simulink model "s06_sig_template"  (R2025a)
settings: Solver=ode4  StartTime=0.0  StopTime=inf  FixedStep=P_sim_dt  RelTol=1e-3  EnableMultiTasking=on
InitFcn:
  | s06_data;
values from neighbouring files (symbols this model uses):
  CarInputsCmdForward = uint8(1)    [i01_data.m]
  ManeuverTypePark = uint8(1)    [i01_data.m]
  ManeuverTypePathFollow = uint8(3)    [i01_data.m]
  P_c_locate_problist = ones(P_car_cnt, 1, 'single')    [s06_data.m]
  P_cpseq = Simulink.Bus.createMATLABStruct('CHECKPOINTSEQUENCEMSG', [])    [i01_data.m]
  P_display_dt = 50e-3    (= 0.05)    [s06_data.m]
  P_dt = 25e-3    (= 0.025)    [s06_data.m]
  P_p_deltan_max = 1    [d01_data.m]    (also in d71_data.m = 0.93)
  P_p_deltan_min = -P_p_deltan_max    (= -1)    [d01_data.m]    (also in d71_data.m = -0.93)
  P_p_un_max = 1    [d01_data.m]    (also in d71_data.m = 0.2)
  P_p_un_min = -P_p_un_max    (= -1)    [d01_data.m]    (also in d71_data.m = -0.2)
  P_p_xvec0 = [ P_p_v0; P_p_s10; P_p_s20; P_p_psi0; 0; 0; 0 ]    [d01_data.m]    (also in d71_data.m)
  P_p_xvec1 = [ P_p_v0; P_p_s11; P_p_s21; P_p_psi1; 0; 0; 0 ]    [d01_data.m]    (also in d71_data.m)
  P_vfilter = single([ 0.0 0.0 ... (first row only)    [s06_data.m]
undefined symbols (not defined in the file or in its folder): mbc_car_display, P_p, P_track
libraries: vrlib x2
settings Model: Creator=ftraenkle  LastModifiedBy=ftraenkle
settings SolverCC: AlgebraicLoopSolver=TrustRegion
settings DataIOCC: LimitDataPoints=on  InspectSignalLogs=on  ReturnWorkspaceOutputs=off
settings OptimizationCC: DefaultParameterBehavior=Inlined  EnhancedBackFolding=on  PassReuseOutputArgsAs=Individual arguments  ExpressionDepthLimit=2147483647.0  ZeroExternalMemoryAtStartup=off  ZeroInternalMemoryAtStartup=off  OptimizeBlockOrder=speed  DifferentSizesBufferReuse=on  OptimizationCustomize=off  EfficientTunableParamExpr=on
settings DebuggingCC: MergeDetectMultiDrivingBlocksExec=none  SolverPrmCheckMsg=warning  ParameterTunabilityLossMsg=error  UnconnectedInputMsg=warning  UnconnectedOutputMsg=warning  UnconnectedLineMsg=warning  BusObjectLabelMismatch=error  AllowSymbolicDim=off  StateNameClashWarn=warning  SFUnexpectedBacktrackingDiag=warning  SFNoUnconditionalDefaultTransitionDiag=warning  SFExecutionAtInitializationDiag=none  ArithmeticOperatorsInVariantConditions=warning
settings HardwareCC: ProdBitPerLong=64.0  ProdHWDeviceType=Intel->x86-64 (Linux 64)
settings ModelReferenceCC: EnableRefExpFcnMdlSchedulingChecks=on  PropagateSignalLabelsOutOfModel=off
settings SFSimCC: SimUseLocalCustomCode=off  CustomCodeUndefinedFunction=UseInterfaceOnly
settings RTWCC: SystemTargetFile=ert.tlc  GenCodeOnly=on  PackageGeneratedCodeAndArtifacts=on  PackageName=d1.zip  TemplateMakefile=ert_default_tmf  GenerateReport=on  RTWUseLocalCustomCode=off  IncludeHyperlinkInReport=on  GenerateTraceInfo=on  GenerateTraceReportEml=on  GPUComputeCapability=3.5  DLArmComputeVersion=19.05  Description=Embedded Coder
settings CodeAppCC: ForceParamTrailComments=on  IgnoreCustomStorageClasses=off  OperatorAnnotations=on  SimulinkDataObjDesc=on  SFDataObjDesc=on  InsertBlockDesc=on
settings ERTTargetCC: ExtModeTransport=0.0  ExtModeStaticAlloc=off  ExtModeMexFile=ext_comm  ExtModeIntrfLevel=Level1  RootIOFormat=Structure reference  ERTCustomFileTemplate=example_file_process.tlc  DynamicArrayContainerType=coder::array  TargetLangStandard=C99 (ISO)  SupportVariableSizeSignals=on
settings ConfigComp: CovMetricSettings=dw  CovSaveCumulativeToWorkspaceVar=on  CovSaveSingleToWorkspaceVar=on  CovExternalEMLEnable=off

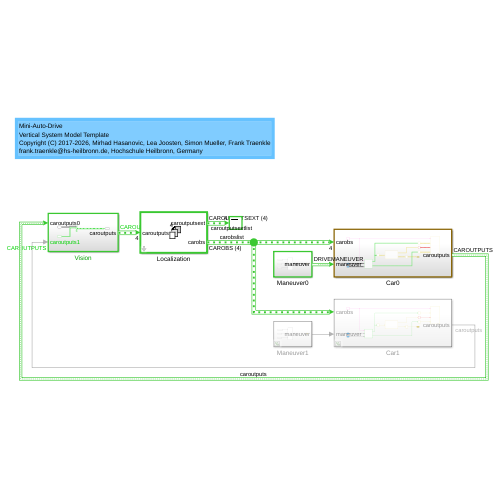
[thumbnail: Simulink's stored preview of the top-level diagram]
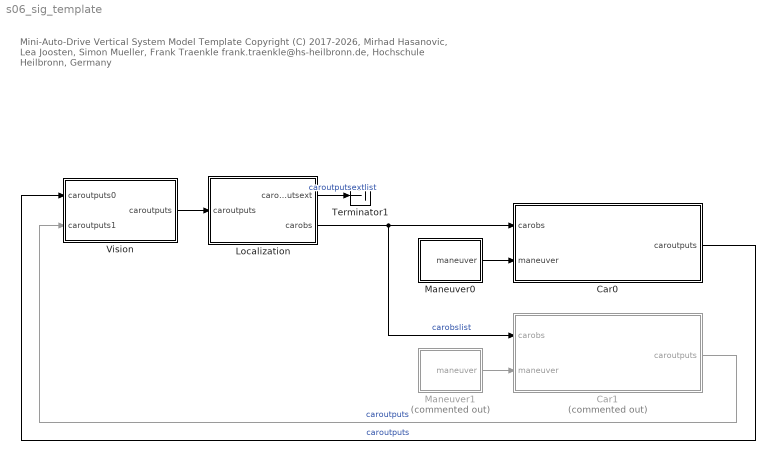
== system s06_sig_template ==
  note: Mini-Auto-Drive
      | Vertical System Model Template
      | Copyright (C) 2017-2026, Mirhad Hasanovic, Lea Joosten, Simon Mueller, Frank Traenkle
      | frank.traenkle@hs-heilbronn.de, Hochschule Heilbronn, Germany
  Car0 : Subsystem
  Car1 : Subsystem  Commented=on
  Localization : Subsystem  TreatAsAtomicUnit=on  mask{P_mask_problist=P_c_locate_problist}
      mask prompts: P_mask_problist "Locate Probability"
  Maneuver0 : Subsystem
  Maneuver1 : Subsystem  Commented=on
  Terminator1 : Terminator
  Vision : Subsystem
  wires:
  Car0/1(caroutputs) -> Vision/1(caroutputs0)  "caroutputs"
  Localization/2(carobs) -> Car1/1(carobs), Car0/1(carobs)  "carobslist"
  Vision/1(caroutputs) -> Localization/1(caroutputs)
  Car1/1(caroutputs) -> Vision/2(caroutputs1)  "caroutputs"
  Maneuver0/1(maneuver) -> Car0/2(maneuver)
  Maneuver1/1(maneuver) -> Car1/2(maneuver)
  Localization/1(caroutputsext) -> Terminator1/1  "caroutputsextlist"

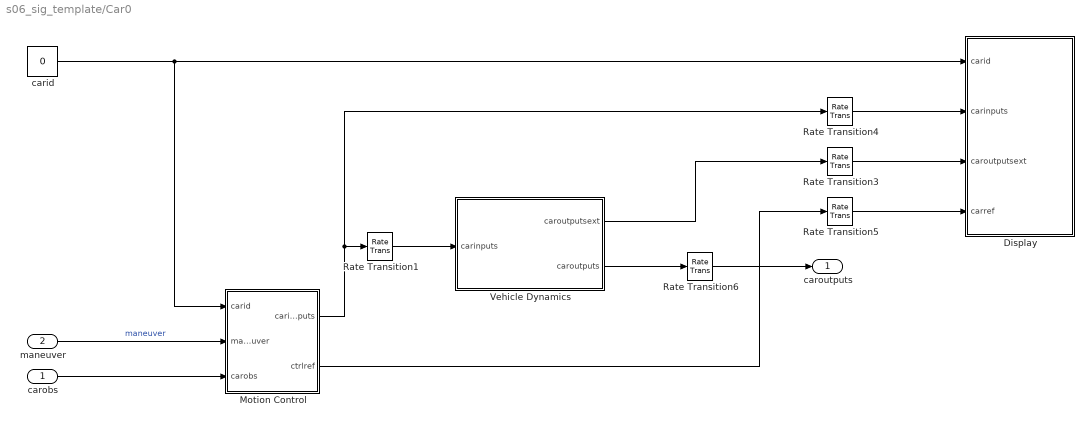
== system s06_sig_template/Car0 ==
  carobs : Inport  OutDataTypeStr=Bus: CAROBS
  maneuver : Inport  Port=2
  Display : Subsystem  TreatAsAtomicUnit=on  SystemSampleTime=P_display_dt
  Motion Control : Subsystem  TreatAsAtomicUnit=on  SystemSampleTime=P_dt
  Rate Transition1 : RateTransition  Integrity=off
  Rate Transition{3..6} (4 alike) : RateTransition
  Vehicle Dynamics : Subsystem  mask{P_mask_vec0=P_p_xvec0, P_mask_p=P_p(1)}
      mask prompts: P_mask_vec0 "Initial value"; P_mask_p "Parameters"
  carid : Constant  Value=0
  caroutputs : Outport  OutDataTypeStr=Bus: CAROUTPUTS
  wires:
  Vehicle Dynamics/1(caroutputsext) -> Rate Transition3/1
  Rate Transition5/1 -> Display/4(carref)
  Rate Transition3/1 -> Display/3(caroutputsext)
  Rate Transition4/1 -> Display/2(carinputs)
  Rate Transition1/1 -> Vehicle Dynamics/1(carinputs)
  Vehicle Dynamics/2(caroutputs) -> Rate Transition6/1
  Rate Transition6/1 -> caroutputs/1
  carid/1 -> Motion Control/1(carid), Display/1(carid)
  Motion Control/1(carinputs) -> Rate Transition4/1, Rate Transition1/1
  Motion Control/2(ctrlref) -> Rate Transition5/1
  carobs/1 -> Motion Control/3(carobs)
  maneuver/1 -> Motion Control/2(maneuver)  "maneuver"

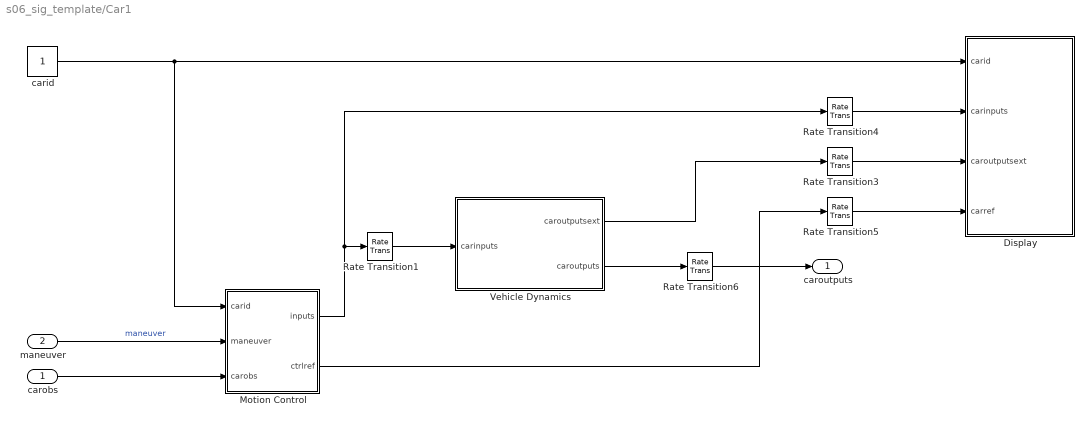
== system s06_sig_template/Car1 ==
  carobs : Inport  OutDataTypeStr=Bus: CAROBS
  maneuver : Inport  Port=2
  Display : Subsystem  TreatAsAtomicUnit=on  SystemSampleTime=P_display_dt
  Motion Control : Subsystem  TreatAsAtomicUnit=on  SystemSampleTime=P_dt
  Rate Transition{1,3..6} (5 alike) : RateTransition
  Vehicle Dynamics : Subsystem  mask{P_mask_vec0=P_p_xvec1, P_mask_p=P_p(1)}
      mask prompts: P_mask_vec0 "Initial value"; P_mask_p "Parameters"
  carid : Constant
  caroutputs : Outport  OutDataTypeStr=Bus: CAROUTPUTS
  wires:
  Vehicle Dynamics/1(caroutputsext) -> Rate Transition3/1
  Rate Transition5/1 -> Display/4(carref)
  Rate Transition3/1 -> Display/3(caroutputsext)
  Rate Transition4/1 -> Display/2(carinputs)
  Rate Transition1/1 -> Vehicle Dynamics/1(carinputs)
  Vehicle Dynamics/2(caroutputs) -> Rate Transition6/1
  Rate Transition6/1 -> caroutputs/1
  carid/1 -> Motion Control/1(carid), Display/1(carid)
  Motion Control/1(inputs) -> Rate Transition4/1, Rate Transition1/1
  Motion Control/2(ctrlref) -> Rate Transition5/1
  carobs/1 -> Motion Control/3(carobs)
  maneuver/1 -> Motion Control/2(maneuver)  "maneuver"

== system s06_sig_template/Localization ==
  caroutputs : Inport  Partition=on  PartitionDimension=1  PartitionWidth=1  PartitionOffset=0
  Constant : Constant  Value=true
  For Each : ForEach  DisableCoverage=on  IterateSubsysMaskParameter=on
  Locate : Subsystem
  caroutputsext : Outport  ConcatenationDimension=1
  carobs : Outport  Port=2  ConcatenationDimension=1
  wires:
  Locate/1(caroutputsext) -> caroutputsext/1
  Constant/1 -> Locate/Enable
  caroutputs/1 -> Locate/1(caroutputs)
  Locate/2(carobs) -> carobs/1

== system s06_sig_template/Maneuver0 ==
  Constant : Constant  Value=ManeuverTypePark
  Constant1 : Constant  Value=single(0.5)
  Constant2 : Constant  Value=single(2.0)
  Create Maneuver : MATLAB Function  TreatAsAtomicUnit=on
  maneuver : Outport
  wires:
  Constant/1 -> Create Maneuver/1(type)
  Constant1/1 -> Create Maneuver/2(vmax)
  Constant2/1 -> Create Maneuver/3(xref)
  Create Maneuver/1(maneuver) -> maneuver/1  "maneuver"

== system s06_sig_template/Maneuver1 ==
  Constant : Constant  Value=ManeuverTypePathFollow
  Constant1 : Constant  Value=single(0.5)
  Constant2 : Constant  Value=single(1.0)
  Create Maneuver : MATLAB Function  TreatAsAtomicUnit=on
  maneuver : Outport
  wires:
  Create Maneuver/1(maneuver) -> maneuver/1  "maneuver"
  Constant2/1 -> Create Maneuver/3(xref)
  Constant1/1 -> Create Maneuver/2(vmax)
  Constant/1 -> Create Maneuver/1(type)

== system s06_sig_template/Vision ==
  caroutputs0 : Inport  OutDataTypeStr=Bus:CAROUTPUTS
  caroutputs1 : Inport  Port=2  OutDataTypeStr=Bus:CAROUTPUTS
  Vector Concatenate : Concatenate  NumInputs=P_car_cnt
  caroutputs : Outport  OutDataTypeStr=Bus:CAROUTPUTS
  wires:
  Vector Concatenate/1 -> caroutputs/1  "caroutputs"
  caroutputs0/1 -> Vector Concatenate/1
  caroutputs1/1 -> Vector Concatenate/2

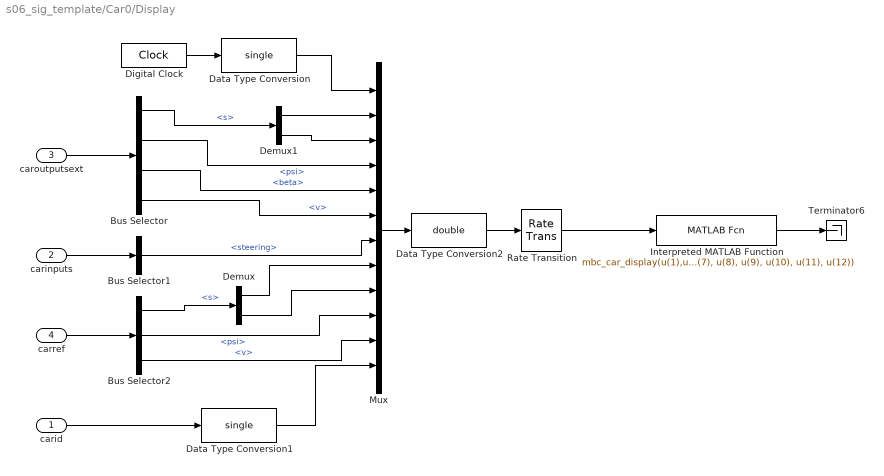
== system s06_sig_template/Car0/Display ==
  carid : Inport
  carinputs : Inport  Port=2
  caroutputsext : Inport  Port=3
  carref : Inport  Port=4
  Bus Selector : BusSelector  OutputSignals=s,psi,beta,v
  Bus Selector1 : BusSelector  OutputSignals=steering
  Bus Selector2 : BusSelector  OutputSignals=s,psi,v
  Data Type Conversion : DataTypeConversion  OutDataTypeStr=single  SaturateOnIntegerOverflow=off  RndMeth=Floor
  Data Type Conversion1 : DataTypeConversion  OutDataTypeStr=single  SaturateOnIntegerOverflow=off  RndMeth=Floor
  Data Type Conversion2 : DataTypeConversion  OutDataTypeStr=double  SaturateOnIntegerOverflow=off  RndMeth=Floor
  Demux : Demux  Outputs=2
  Demux1 : Demux  Outputs=2
  Digital Clock : DigitalClock  SampleTime=-1
  Interpreted MATLAB Function : MATLABFcn  MATLABFcn=mbc_car_display(u(1),u(2),u(3),u(4),u(5), u(6), u(7), u(8), u(9), u(10), u(11), u(12))
  Mux : Mux  Inputs=12
  Rate Transition : RateTransition  OutPortSampleTime=P_display_dt
  Terminator6 : Terminator
  wires:
  caroutputsext/1 -> Bus Selector/1
  Interpreted MATLAB Function/1 -> Terminator6/1
  Mux/1 -> Data Type Conversion2/1
  Rate Transition/1 -> Interpreted MATLAB Function/1
  Digital Clock/1 -> Data Type Conversion/1
  Bus Selector/2 -> Mux/4  "<psi>"
  carinputs/1 -> Bus Selector1/1
  Bus Selector1/1 -> Mux/7  "<steering>"
  Bus Selector/3 -> Mux/5  "<beta>"
  Bus Selector/4 -> Mux/6  "<v>"
  carref/1 -> Bus Selector2/1
  Bus Selector2/3 -> Mux/11  "<v>"
  Bus Selector2/2 -> Mux/10  "<psi>"
  Bus Selector2/1 -> Demux/1  "<s>"
  carid/1 -> Data Type Conversion1/1
  Data Type Conversion/1 -> Mux/1
  Data Type Conversion1/1 -> Mux/12
  Data Type Conversion2/1 -> Rate Transition/1
  Demux/1 -> Mux/8
  Demux/2 -> Mux/9
  Bus Selector/1 -> Demux1/1  "<s>"
  Demux1/1 -> Mux/2
  Demux1/2 -> Mux/3

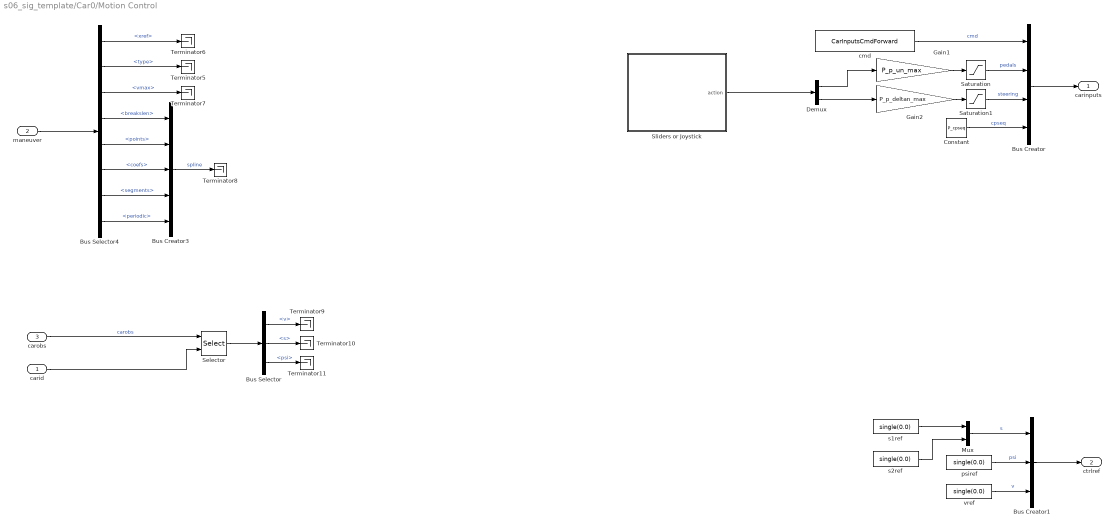
== system s06_sig_template/Car0/Motion Control ==
  carid : Inport
  maneuver : Inport  Port=2
  carobs : Inport  Port=3
  Bus Creator : BusCreator  Inputs=4  OutDataTypeStr=Bus: CARINPUTS  NonVirtualBus=on
  Bus Creator1 : BusCreator  Inputs=3  OutDataTypeStr=Bus: CTRLREFERENCE  NonVirtualBus=on
  Bus Creator3 : BusCreator  Inputs=5  OutDataTypeStr=Bus: SPLINE
  Bus Selector : BusSelector  OutputSignals=v,s,psi
  Bus Selector4 : BusSelector  OutputSignals=xref,type,vmax,breakslen,points,coefs,segments,periodic
  Constant : Constant  Value=P_cpseq  OutDataTypeStr=Bus: CHECKPOINTSEQUENCEMSG
  Demux : Demux  Outputs=2
  Gain1 : Gain  Gain=P_p_un_max
  Gain2 : Gain  Gain=P_p_deltan_max
  Mux : Mux  Inputs=2
  Saturation : Saturate  UpperLimit=P_p_un_max  LowerLimit=P_p_un_min
  Saturation1 : Saturate  UpperLimit=P_p_deltan_max  LowerLimit=P_p_deltan_min
  Selector : Selector  IndexMode=Zero-based  InputPortWidth=P_car_cnt  IndexOptions=Index vector (port)  Indices=0  OutputSizes=1
  Sliders or Joystick : Subsystem  Variant=on  VariantControlMode=label  LabelModeActiveChoice=true
  Terminator{5..11} (7 alike) : Terminator
  cmd : Constant  Value=CarInputsCmdForward
  psiref : Constant  Value=single(0.0)
  s1ref : Constant  Value=single(0.0)
  s2ref : Constant  Value=single(0.0)
  vref : Constant  Value=single(0.0)
  carinputs : Outport  VectorParamsAs1DForOutWhenUnconnected=off
  ctrlref : Outport  Port=2  VectorParamsAs1DForOutWhenUnconnected=off
  wires:
  Bus Creator1/1 -> ctrlref/1
  vref/1 -> Bus Creator1/3  "v"
  Bus Selector/2 -> Terminator10/1  "<s>"
  Mux/1 -> Bus Creator1/1  "s"
  Bus Selector4/7 -> Bus Creator3/4  "<segments>"
  Bus Selector4/5 -> Bus Creator3/2  "<points>"
  Bus Selector4/6 -> Bus Creator3/3  "<coefs>"
  Bus Selector4/8 -> Bus Creator3/5  "<periodic>"
  Bus Selector4/2 -> Terminator5/1  "<type>"
  Bus Selector4/4 -> Bus Creator3/1  "<breakslen>"
  maneuver/1 -> Bus Selector4/1
  carid/1 -> Selector/2
  carobs/1 -> Selector/1  "carobs"
  Selector/1 -> Bus Selector/1
  Bus Selector4/1 -> Terminator6/1  "<xref>"
  Bus Selector4/3 -> Terminator7/1  "<vmax>"
  Bus Creator3/1 -> Terminator8/1  "spline"
  Bus Selector/1 -> Terminator9/1  "<v>"
  Bus Selector/3 -> Terminator11/1  "<psi>"
  s1ref/1 -> Mux/1
  s2ref/1 -> Mux/2
  psiref/1 -> Bus Creator1/2  "psi"
  Saturation/1 -> Bus Creator/2  "pedals"
  Demux/1 -> Gain1/1
  Constant/1 -> Bus Creator/4  "cpseq"
  Bus Creator/1 -> carinputs/1
  cmd/1 -> Bus Creator/1  "cmd"
  Gain1/1 -> Saturation/1
  Saturation1/1 -> Bus Creator/3  "steering"
  Sliders or Joystick/1(action) -> Demux/1
  Demux/2 -> Gain2/1
  Gain2/1 -> Saturation1/1

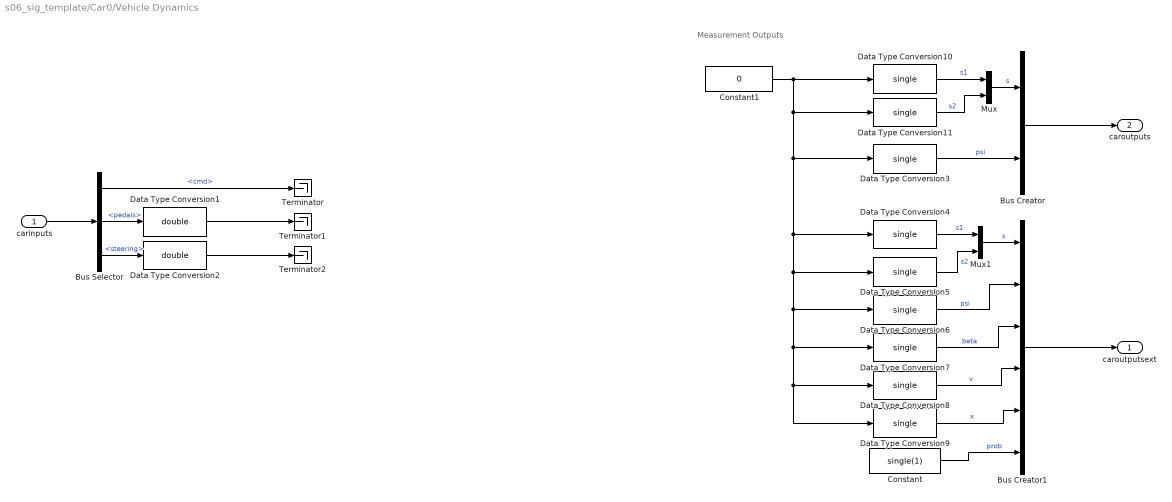
== system s06_sig_template/Car0/Vehicle Dynamics ==
  note: Measurement Outputs
  carinputs : Inport
  Bus Creator : BusCreator  Inputs=2  OutDataTypeStr=Bus: CAROUTPUTS  NonVirtualBus=on
  Bus Creator1 : BusCreator  Inputs=6  OutDataTypeStr=Bus: CAROUTPUTSEXT  NonVirtualBus=on
  Bus Selector : BusSelector  OutputSignals=cmd,pedals,steering
  Constant : Constant  Value=single(1)
  Constant1 : Constant  Value=0
  Data Type Conversion1 : DataTypeConversion  OutDataTypeStr=double  SaturateOnIntegerOverflow=off  RndMeth=Floor
  Data Type Conversion{3..11} (9 alike) : DataTypeConversion  OutDataTypeStr=single  SaturateOnIntegerOverflow=off  RndMeth=Floor
  Data Type Conversion2 : DataTypeConversion  OutDataTypeStr=double  SaturateOnIntegerOverflow=off  RndMeth=Floor
  Mux : Mux  Inputs=2
  Mux1 : Mux  Inputs=2
  Terminator : Terminator
  Terminator1 : Terminator
  Terminator2 : Terminator
  caroutputsext : Outport  OutDataTypeStr=Bus: CAROUTPUTSEXT  VectorParamsAs1DForOutWhenUnconnected=off
  caroutputs : Outport  Port=2  OutDataTypeStr=Bus: CAROUTPUTS  VectorParamsAs1DForOutWhenUnconnected=off
  wires:
  carinputs/1 -> Bus Selector/1
  Bus Selector/2 -> Data Type Conversion1/1  "<pedals>"
  Bus Selector/3 -> Data Type Conversion2/1  "<steering>"
  Bus Creator/1 -> caroutputs/1
  Bus Creator1/1 -> caroutputsext/1
  Bus Selector/1 -> Terminator/1  "<cmd>"
  Data Type Conversion1/1 -> Terminator1/1
  Data Type Conversion2/1 -> Terminator2/1
  Constant1/1 -> Data Type Conversion9/1, Data Type Conversion8/1, Data Type Conversion7/1, Data Type Conversion6/1, Data Type Conversion5/1, Data Type Conversion4/1, Data Type Conversion3/1, Data Type Conversion11/1, Data Type Conversion10/1
  Mux1/1 -> Bus Creator1/1  "s"
  Data Type Conversion5/1 -> Mux1/2  "s2"
  Data Type Conversion4/1 -> Mux1/1  "s1"
  Mux/1 -> Bus Creator/1  "s"
  Data Type Conversion9/1 -> Bus Creator1/5  "x"
  Data Type Conversion8/1 -> Bus Creator1/4  "v"
  Data Type Conversion7/1 -> Bus Creator1/3  "beta"
  Data Type Conversion6/1 -> Bus Creator1/2  "psi"
  Data Type Conversion3/1 -> Bus Creator/2  "psi"
  Data Type Conversion11/1 -> Mux/2  "s2"
  Data Type Conversion10/1 -> Mux/1  "s1"
  Constant/1 -> Bus Creator1/6  "prob"

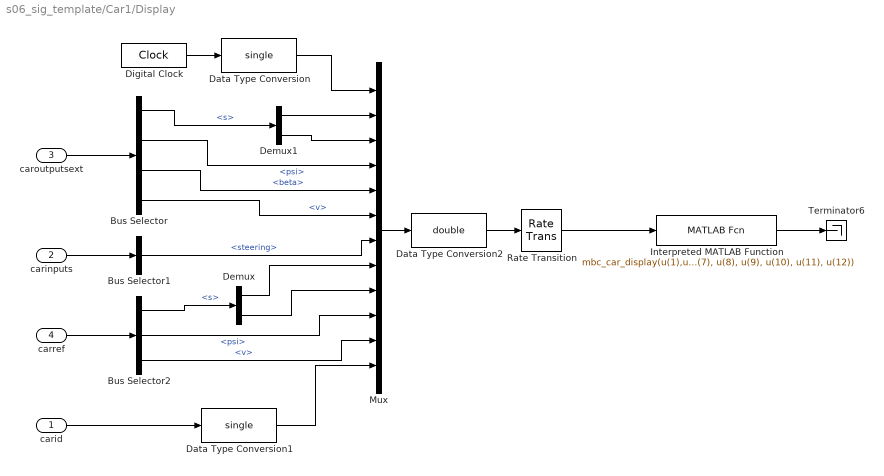
== system s06_sig_template/Car1/Display ==
  carid : Inport
  carinputs : Inport  Port=2
  caroutputsext : Inport  Port=3
  carref : Inport  Port=4
  Bus Selector : BusSelector  OutputSignals=s,psi,beta,v
  Bus Selector1 : BusSelector  OutputSignals=steering
  Bus Selector2 : BusSelector  OutputSignals=s,psi,v
  Data Type Conversion : DataTypeConversion  OutDataTypeStr=single  SaturateOnIntegerOverflow=off  RndMeth=Floor
  Data Type Conversion1 : DataTypeConversion  OutDataTypeStr=single  SaturateOnIntegerOverflow=off  RndMeth=Floor
  Data Type Conversion2 : DataTypeConversion  OutDataTypeStr=double  SaturateOnIntegerOverflow=off  RndMeth=Floor
  Demux : Demux  Outputs=2
  Demux1 : Demux  Outputs=2
  Digital Clock : DigitalClock  SampleTime=-1
  Interpreted MATLAB Function : MATLABFcn  MATLABFcn=mbc_car_display(u(1),u(2),u(3),u(4),u(5), u(6), u(7), u(8), u(9), u(10), u(11), u(12))
  Mux : Mux  Inputs=12
  Rate Transition : RateTransition  OutPortSampleTime=P_display_dt
  Terminator6 : Terminator
  wires:
  caroutputsext/1 -> Bus Selector/1
  Interpreted MATLAB Function/1 -> Terminator6/1
  Mux/1 -> Data Type Conversion2/1
  Rate Transition/1 -> Interpreted MATLAB Function/1
  Digital Clock/1 -> Data Type Conversion/1
  Bus Selector/2 -> Mux/4  "<psi>"
  carinputs/1 -> Bus Selector1/1
  Bus Selector1/1 -> Mux/7  "<steering>"
  Bus Selector/3 -> Mux/5  "<beta>"
  Bus Selector/4 -> Mux/6  "<v>"
  carref/1 -> Bus Selector2/1
  Bus Selector2/3 -> Mux/11  "<v>"
  Bus Selector2/2 -> Mux/10  "<psi>"
  Bus Selector2/1 -> Demux/1  "<s>"
  carid/1 -> Data Type Conversion1/1
  Data Type Conversion/1 -> Mux/1
  Data Type Conversion1/1 -> Mux/12
  Data Type Conversion2/1 -> Rate Transition/1
  Demux/1 -> Mux/8
  Demux/2 -> Mux/9
  Bus Selector/1 -> Demux1/1  "<s>"
  Demux1/1 -> Mux/2
  Demux1/2 -> Mux/3

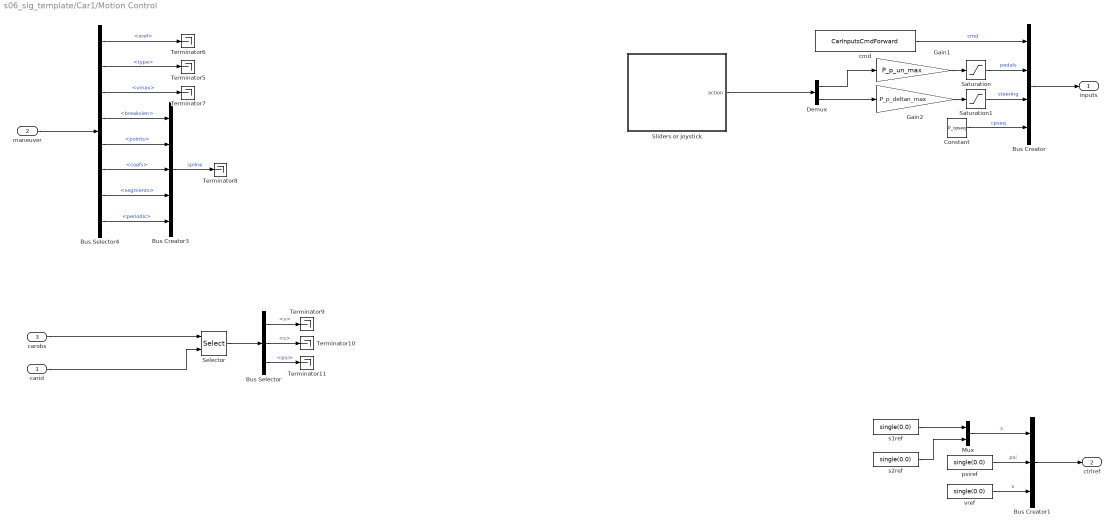
== system s06_sig_template/Car1/Motion Control ==
  carid : Inport
  maneuver : Inport  Port=2
  carobs : Inport  Port=3
  Bus Creator : BusCreator  Inputs=4  OutDataTypeStr=Bus: CARINPUTS  NonVirtualBus=on
  Bus Creator1 : BusCreator  Inputs=3  OutDataTypeStr=Bus: CTRLREFERENCE  NonVirtualBus=on
  Bus Creator3 : BusCreator  Inputs=5  OutDataTypeStr=Bus: SPLINE
  Bus Selector : BusSelector  OutputSignals=v,s,psi
  Bus Selector4 : BusSelector  OutputSignals=xref,type,vmax,breakslen,points,coefs,segments,periodic
  Constant : Constant  Value=P_cpseq  OutDataTypeStr=Bus: CHECKPOINTSEQUENCEMSG
  Demux : Demux  Outputs=2
  Gain1 : Gain  Gain=P_p_un_max
  Gain2 : Gain  Gain=P_p_deltan_max
  Mux : Mux  Inputs=2
  Saturation : Saturate  UpperLimit=P_p_un_max  LowerLimit=P_p_un_min
  Saturation1 : Saturate  UpperLimit=P_p_deltan_max  LowerLimit=P_p_deltan_min
  Selector : Selector  IndexMode=Zero-based  InputPortWidth=P_car_cnt  IndexOptions=Index vector (port)  Indices=0  OutputSizes=1
  Sliders or Joystick : Subsystem  Variant=on  VariantControlMode=label  LabelModeActiveChoice=true
  Terminator{5..11} (7 alike) : Terminator
  cmd : Constant  Value=CarInputsCmdForward
  psiref : Constant  Value=single(0.0)
  s1ref : Constant  Value=single(0.0)
  s2ref : Constant  Value=single(0.0)
  vref : Constant  Value=single(0.0)
  inputs : Outport  VectorParamsAs1DForOutWhenUnconnected=off
  ctrlref : Outport  Port=2  VectorParamsAs1DForOutWhenUnconnected=off
  wires:
  Bus Creator1/1 -> ctrlref/1
  vref/1 -> Bus Creator1/3  "v"
  Bus Selector/2 -> Terminator10/1  "<s>"
  Mux/1 -> Bus Creator1/1  "s"
  Bus Selector4/7 -> Bus Creator3/4  "<segments>"
  Bus Selector4/5 -> Bus Creator3/2  "<points>"
  Bus Selector4/6 -> Bus Creator3/3  "<coefs>"
  Bus Selector4/8 -> Bus Creator3/5  "<periodic>"
  Bus Selector4/2 -> Terminator5/1  "<type>"
  Bus Selector4/4 -> Bus Creator3/1  "<breakslen>"
  maneuver/1 -> Bus Selector4/1
  carid/1 -> Selector/2
  carobs/1 -> Selector/1
  Selector/1 -> Bus Selector/1
  Bus Selector4/1 -> Terminator6/1  "<xref>"
  Bus Selector4/3 -> Terminator7/1  "<vmax>"
  Bus Creator3/1 -> Terminator8/1  "spline"
  Bus Selector/1 -> Terminator9/1  "<v>"
  Bus Selector/3 -> Terminator11/1  "<psi>"
  s1ref/1 -> Mux/1
  s2ref/1 -> Mux/2
  psiref/1 -> Bus Creator1/2  "psi"
  Saturation/1 -> Bus Creator/2  "pedals"
  Demux/1 -> Gain1/1
  Constant/1 -> Bus Creator/4  "cpseq"
  Bus Creator/1 -> inputs/1
  cmd/1 -> Bus Creator/1  "cmd"
  Gain1/1 -> Saturation/1
  Saturation1/1 -> Bus Creator/3  "steering"
  Sliders or Joystick/1(action) -> Demux/1
  Demux/2 -> Gain2/1
  Gain2/1 -> Saturation1/1

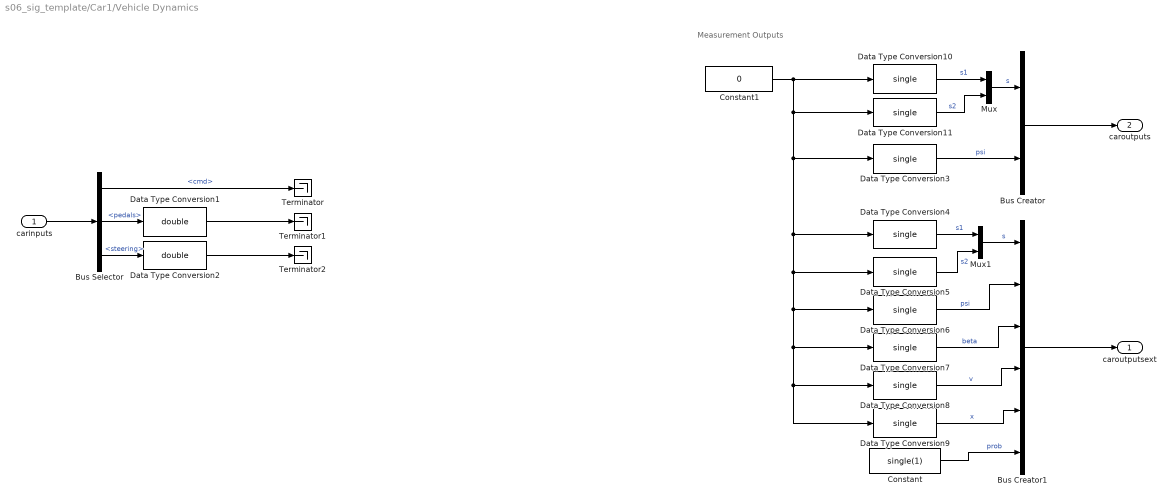
== system s06_sig_template/Car1/Vehicle Dynamics ==
  note: Measurement Outputs
  carinputs : Inport
  Bus Creator : BusCreator  Inputs=2  OutDataTypeStr=Bus: CAROUTPUTS  NonVirtualBus=on
  Bus Creator1 : BusCreator  Inputs=6  OutDataTypeStr=Bus: CAROUTPUTSEXT  NonVirtualBus=on
  Bus Selector : BusSelector  OutputSignals=cmd,pedals,steering
  Constant : Constant  Value=single(1)
  Constant1 : Constant  Value=0
  Data Type Conversion1 : DataTypeConversion  OutDataTypeStr=double  SaturateOnIntegerOverflow=off  RndMeth=Floor
  Data Type Conversion{3..11} (9 alike) : DataTypeConversion  OutDataTypeStr=single  SaturateOnIntegerOverflow=off  RndMeth=Floor
  Data Type Conversion2 : DataTypeConversion  OutDataTypeStr=double  SaturateOnIntegerOverflow=off  RndMeth=Floor
  Mux : Mux  Inputs=2
  Mux1 : Mux  Inputs=2
  Terminator : Terminator
  Terminator1 : Terminator
  Terminator2 : Terminator
  caroutputsext : Outport  OutDataTypeStr=Bus: CAROUTPUTSEXT  VectorParamsAs1DForOutWhenUnconnected=off
  caroutputs : Outport  Port=2  OutDataTypeStr=Bus: CAROUTPUTS  VectorParamsAs1DForOutWhenUnconnected=off
  wires:
  carinputs/1 -> Bus Selector/1
  Bus Selector/2 -> Data Type Conversion1/1  "<pedals>"
  Bus Selector/3 -> Data Type Conversion2/1  "<steering>"
  Bus Creator/1 -> caroutputs/1
  Bus Creator1/1 -> caroutputsext/1
  Bus Selector/1 -> Terminator/1  "<cmd>"
  Data Type Conversion1/1 -> Terminator1/1
  Data Type Conversion2/1 -> Terminator2/1
  Constant1/1 -> Data Type Conversion9/1, Data Type Conversion8/1, Data Type Conversion7/1, Data Type Conversion6/1, Data Type Conversion5/1, Data Type Conversion4/1, Data Type Conversion3/1, Data Type Conversion11/1, Data Type Conversion10/1
  Mux1/1 -> Bus Creator1/1  "s"
  Data Type Conversion5/1 -> Mux1/2  "s2"
  Data Type Conversion4/1 -> Mux1/1  "s1"
  Mux/1 -> Bus Creator/1  "s"
  Data Type Conversion9/1 -> Bus Creator1/5  "x"
  Data Type Conversion8/1 -> Bus Creator1/4  "v"
  Data Type Conversion7/1 -> Bus Creator1/3  "beta"
  Data Type Conversion6/1 -> Bus Creator1/2  "psi"
  Data Type Conversion3/1 -> Bus Creator/2  "psi"
  Data Type Conversion11/1 -> Mux/2  "s2"
  Data Type Conversion10/1 -> Mux/1  "s1"
  Constant/1 -> Bus Creator1/6  "prob"

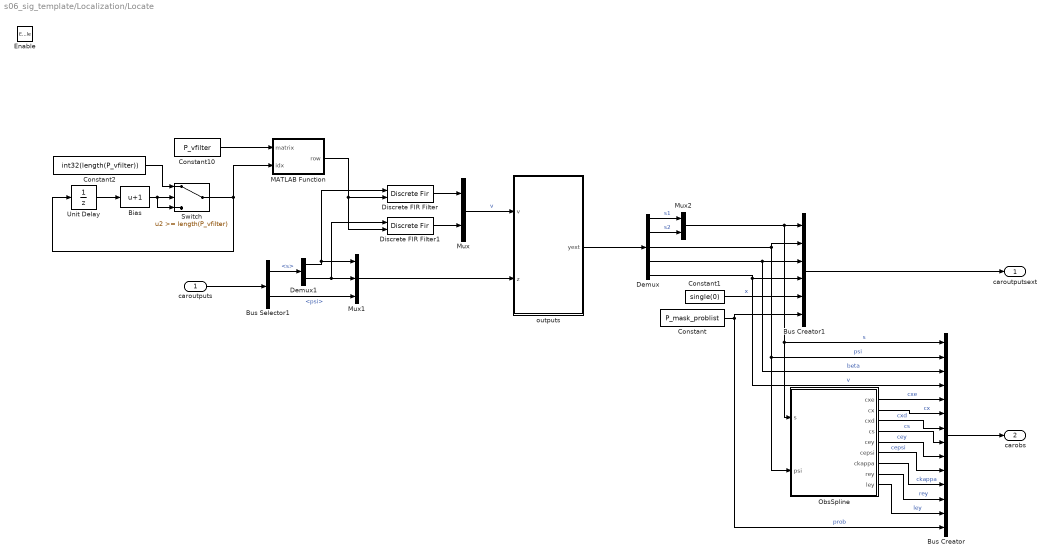
== system s06_sig_template/Localization/Locate ==
  caroutputs : Inport
  Enable : EnablePort
  Bias : Bias  Bias=1  SaturateOnIntegerOverflow=off
  Bus Creator : BusCreator  Inputs=14  OutDataTypeStr=Bus: CAROBS  NonVirtualBus=on
  Bus Creator1 : BusCreator  Inputs=6  OutDataTypeStr=Bus: CAROUTPUTSEXT  NonVirtualBus=on
  Bus Selector1 : BusSelector  OutputSignals=s,psi
  Constant : Constant  Value=P_mask_problist
  Constant1 : Constant  Value=single(0)
  Constant10 : Constant  Value=P_vfilter
  Constant2 : Constant  Value=int32(length(P_vfilter))
  Demux : Demux  Outputs=5
  Demux1 : Demux  Outputs=2
  Discrete FIR Filter : DiscreteFir  CoefSource=Input port
      settings: InputPortMap=u0,u1
  Discrete FIR Filter1 : DiscreteFir  CoefSource=Input port
      settings: InputPortMap=u0,u1
  MATLAB Function : MATLAB Function  TreatAsAtomicUnit=on
  Mux : Mux  Inputs=2
  Mux1 : Mux  Inputs=3
  Mux2 : Mux  Inputs=2
  ObsSpline : Subsystem
  Switch : Switch  Threshold=length(P_vfilter)  SaturateOnIntegerOverflow=off  InputSameDT=off
  Unit Delay : UnitDelay  InitialCondition=int32(0)  SampleTime=-1  HasFrameUpgradeWarning=on
  outputs : MATLAB Function  TreatAsAtomicUnit=on  SystemSampleTime=P_dt
  caroutputsext : Outport
  carobs : Outport  Port=2
  wires:
  Mux1/1 -> outputs/2(z)
  Bus Selector1/2 -> Mux1/3  "<psi>"
  MATLAB Function/1(row) -> Discrete FIR Filter1/2, Discrete FIR Filter/2
  Discrete FIR Filter1/1 -> Mux/2
  Discrete FIR Filter/1 -> Mux/1
  Constant/1 -> Bus Creator/14, Bus Creator1/6  "prob"
  Bus Selector1/1 -> Demux1/1  "<s>"
  Demux1/2 -> Discrete FIR Filter1/1, Mux1/2
  Demux/4 -> Bus Creator/3, Bus Creator1/3  "beta"
  Mux2/1 -> ObsSpline/1(s), Bus Creator/1, Bus Creator1/1  "s"
  caroutputs/1 -> Bus Selector1/1
  Constant1/1 -> Bus Creator1/5  "x"
  Demux/1 -> Mux2/1  "s1"
  Demux/2 -> Mux2/2  "s2"
  Demux1/1 -> Discrete FIR Filter/1, Mux1/1
  Bus Creator1/1 -> caroutputsext/1
  Demux/5 -> Bus Creator/4, Bus Creator1/4  "v"
  Mux/1 -> outputs/1(v)  "v"
  outputs/1(yext) -> Demux/1
  Demux/3 -> ObsSpline/2(psi), Bus Creator/2, Bus Creator1/2  "psi"
  Constant10/1 -> MATLAB Function/1(matrix)
  Switch/1 -> Unit Delay/1, MATLAB Function/2(idx)
  Unit Delay/1 -> Bias/1
  Bias/1 -> Switch/3, Switch/2
  Constant2/1 -> Switch/1
  ObsSpline/1(cxe) -> Bus Creator/5  "cxe"
  ObsSpline/2(cx) -> Bus Creator/6  "cx"
  ObsSpline/3(cxd) -> Bus Creator/7  "cxd"
  ObsSpline/5(cey) -> Bus Creator/9  "cey"
  ObsSpline/6(cepsi) -> Bus Creator/10  "cepsi"
  ObsSpline/7(ckappa) -> Bus Creator/11  "ckappa"
  ObsSpline/8(rey) -> Bus Creator/12  "rey"
  ObsSpline/9(ley) -> Bus Creator/13  "ley"
  Bus Creator/1 -> carobs/1
  ObsSpline/4(cs) -> Bus Creator/8  "cs"

== system s06_sig_template/Car0/Motion Control/Sliders or Joystick ==
  note: 1) Add Subsystem or Model blocks as valid variant choices.
      | 2) You cannot connect blocks at this level. At simulation, connectivity is automatically
      | determined, based on the active variant and port name matching.
  Joystick : Subsystem  VariantControl=false
  Sliders : Subsystem  VariantControl=true
  action : Outport

== system s06_sig_template/Car1/Motion Control/Sliders or Joystick ==
  note: 1) Add Subsystem or Model blocks as valid variant choices.
      | 2) You cannot connect blocks at this level. At simulation, connectivity is automatically
      | determined, based on the active variant and port name matching.
  Joystick : Subsystem  VariantControl=false
  Sliders : Subsystem  VariantControl=true
  action : Outport

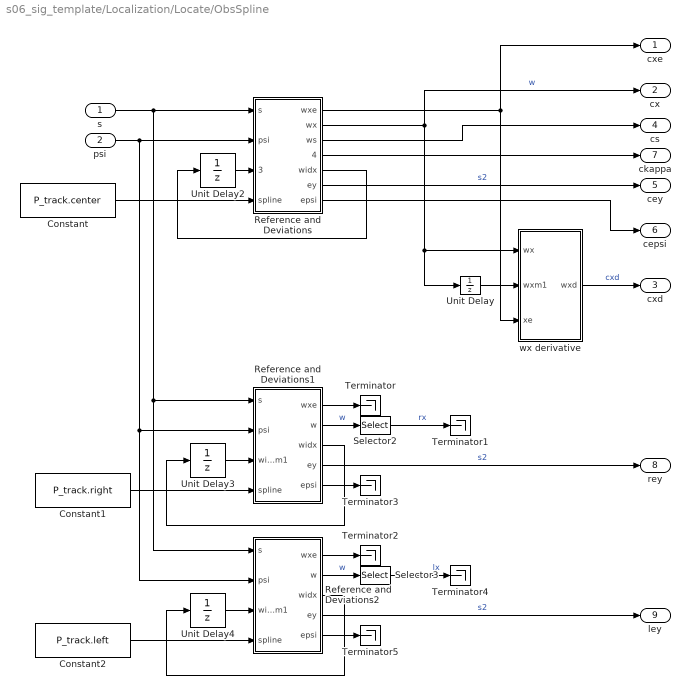
== system s06_sig_template/Localization/Locate/ObsSpline ==
  s : Inport
  psi : Inport  Port=2
  Constant : Constant  Value=P_track.center  OutDataTypeStr=Bus: SPLINE
  Constant1 : Constant  Value=P_track.right  OutDataTypeStr=Bus: SPLINE
  Constant2 : Constant  Value=P_track.left  OutDataTypeStr=Bus: SPLINE
  Reference and Deviations : MATLAB Function  TreatAsAtomicUnit=on
  Reference and Deviations1 : MATLAB Function  TreatAsAtomicUnit=on
  Reference and Deviations2 : MATLAB Function  TreatAsAtomicUnit=on
  Selector2 : Selector  InputPortWidth=5  IndexOptions=Index vector (dialog)  Indices=1  OutputSizes=1
  Selector3 : Selector  InputPortWidth=5  IndexOptions=Index vector (dialog)  Indices=1  OutputSizes=1
  Terminator{,1..5} (6 alike) : Terminator
  Unit Delay : UnitDelay  InitialCondition=-1  SampleTime=-1  HasFrameUpgradeWarning=on
  Unit Delay2 : UnitDelay  InitialCondition=int32(0)  SampleTime=-1  HasFrameUpgradeWarning=on
  Unit Delay3 : UnitDelay  InitialCondition=int32(0)  SampleTime=-1  HasFrameUpgradeWarning=on
  Unit Delay4 : UnitDelay  InitialCondition=int32(0)  SampleTime=-1  HasFrameUpgradeWarning=on
  wx derivative : MATLAB Function  TreatAsAtomicUnit=on
  cxe : Outport
  cx : Outport  Port=2
  cxd : Outport  Port=3
  cs : Outport  Port=4
  cey : Outport  Port=5
  cepsi : Outport  Port=6
  ckappa : Outport  Port=7
  rey : Outport  Port=8
  ley : Outport  Port=9
  wires:
  Reference and Deviations/6(ey) -> cey/1  "s2"
  Unit Delay/1 -> wx derivative/2(wxm1)
  s/1 -> Reference and Deviations2/1(s), Reference and Deviations1/1(s), Reference and Deviations/1(s)
  Unit Delay2/1 -> Reference and Deviations/3(widxkm1)
  Reference and Deviations/5(widx) -> Unit Delay2/1
  psi/1 -> Reference and Deviations2/2(psi), Reference and Deviations1/2(psi), Reference and Deviations/2(psi)
  Constant/1 -> Reference and Deviations/4(spline)
  Reference and Deviations/7(epsi) -> cepsi/1
  Reference and Deviations/2(wx) -> wx derivative/1(wx), Unit Delay/1, cx/1  "w"
  Reference and Deviations/1(wxe) -> wx derivative/3(xe), cxe/1
  wx derivative/1(wxd) -> cxd/1  "cxd"
  Reference and Deviations/4(wkappa) -> ckappa/1
  Unit Delay3/1 -> Reference and Deviations1/3(widxkm1)
  Reference and Deviations1/3(widx) -> Unit Delay3/1
  Reference and Deviations1/1(wxe) -> Terminator/1
  Reference and Deviations1/2(w) -> Selector2/1  "w"
  Reference and Deviations1/4(ey) -> rey/1  "s2"
  Reference and Deviations1/5(epsi) -> Terminator3/1
  Constant1/1 -> Reference and Deviations1/4(spline)
  Unit Delay4/1 -> Reference and Deviations2/3(widxkm1)
  Constant2/1 -> Reference and Deviations2/4(spline)
  Reference and Deviations2/1(wxe) -> Terminator2/1
  Reference and Deviations2/4(ey) -> ley/1  "s2"
  Reference and Deviations2/3(widx) -> Unit Delay4/1
  Reference and Deviations2/5(epsi) -> Terminator5/1
  Reference and Deviations2/2(w) -> Selector3/1  "w"
  Selector2/1 -> Terminator1/1  "rx"
  Selector3/1 -> Terminator4/1  "lx"
  Reference and Deviations/3(ws) -> cs/1

== system s06_sig_template/Car0/Motion Control/Sliders or Joystick/Joystick ==
  Data Type Conversion : DataTypeConversion  OutDataTypeStr=single  SaturateOnIntegerOverflow=off  RndMeth=Floor
  Gain3 : Gain  Gain=-1
  Joystick Input : vrlib/Joystick Input  joyid=1  adjustports=off  forcefeed=off
  Selector1 : Selector  IndexOptions=Index vector (dialog)  Indices=[2 4]  OutputSizes=1
  Terminator : Terminator
  action : Outport
  wires:
  Data Type Conversion/1 -> Selector1/1
  Gain3/1 -> action/1
  Joystick Input/1 -> Data Type Conversion/1
  Selector1/1 -> Gain3/1
  Joystick Input/2 -> Terminator/1

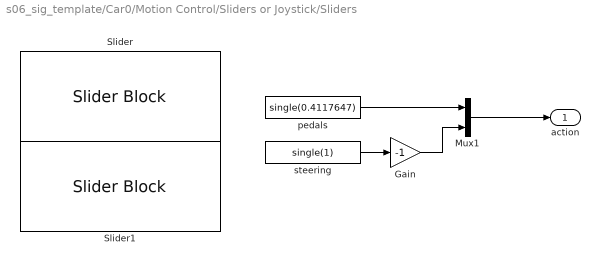
== system s06_sig_template/Car0/Motion Control/Sliders or Joystick/Sliders ==
  Gain : Gain  Gain=-1
  Mux1 : Mux  Inputs=2
  Slider : SliderBlock  ScaleMin=-1  ScaleMax=1
  Slider1 : SliderBlock  ScaleMin=-1  ScaleMax=1
  pedals : Constant  Value=single(0.4117647)  SampleTime=Inf
  steering : Constant  Value=single(1)
  action : Outport
  wires:
  pedals/1 -> Mux1/1
  Gain/1 -> Mux1/2
  Mux1/1 -> action/1
  steering/1 -> Gain/1

== system s06_sig_template/Car1/Motion Control/Sliders or Joystick/Joystick ==
  Data Type Conversion : DataTypeConversion  OutDataTypeStr=single  SaturateOnIntegerOverflow=off  RndMeth=Floor
  Gain3 : Gain  Gain=-1
  Joystick Input : vrlib/Joystick Input  joyid=1  adjustports=off  forcefeed=off
  Selector1 : Selector  IndexOptions=Index vector (dialog)  Indices=[2 4]  OutputSizes=1
  Terminator : Terminator
  action : Outport
  wires:
  Data Type Conversion/1 -> Selector1/1
  Gain3/1 -> action/1
  Joystick Input/1 -> Data Type Conversion/1
  Selector1/1 -> Gain3/1
  Joystick Input/2 -> Terminator/1

== system s06_sig_template/Car1/Motion Control/Sliders or Joystick/Sliders ==
  Gain : Gain  Gain=-1
  Mux1 : Mux  Inputs=2
  Slider : SliderBlock  ScaleMin=-1  ScaleMax=1
  Slider1 : SliderBlock  ScaleMin=-1  ScaleMax=1
  pedals : Constant  Value=single(0.4117647)  SampleTime=Inf
  steering : Constant  Value=single(1)
  action : Outport
  wires:
  pedals/1 -> Mux1/1
  Gain/1 -> Mux1/2
  Mux1/1 -> action/1
  steering/1 -> Gain/1

== matlab function s06_sig_template/Localization/Locate/MATLAB Function ==
  data: matrix input; row output; idx input int32
function row = fcn(matrix, idx)
row = matrix(idx,:);
end

== matlab function s06_sig_template/Localization/Locate/outputs ==
  data: v input; z input; yext output size=5
function yext = outputs(v, z) 
%#codegen

psi = z(3);
vabs = sqrt(v(1)*v(1) + v(2)*v(2));
beta = mod(atan2(v(2), v(1)) - psi, 2*pi);
if beta > pi
    beta = beta - 2*pi;
end
if abs(beta) > 0.5 * pi
    vabs = -vabs;
end

yext = [ ...
    z(1) ; ...
    z(2) ; ...
    psi ; ...
    beta ; ...
    vabs ...
    ];
end

== matlab function s06_sig_template/Localization/Locate/ObsSpline/Reference and Deviations ==
  data: wxe output; s input; psi input; widxkm1 input int32; spline input; P_c_spline_range parameter; wx output; ws output; wkappa output; widx output; ey output; epsi output
function [ wxe, wx, ws, wkappa, widx, ey, epsi ] = fcn(s, psi, widxkm1, spline, P_c_spline_range)
%#codegen
wxe = spline.points(1, spline.breakslen);
if widxkm1 < int32(1)
    % first call
    irangemin = int32(1);
    irangemax = int32(spline.breakslen);
else
    irangemin = widxkm1 - P_c_spline_range;
    irangemax = widxkm1 + P_c_spline_range;
end
[ w , widx ] = mbc_spline_get_reference(s, spline.breakslen, spline.points, spline.coefs, spline.periodic, 0, 0, irangemin, irangemax);
wx = w(1);
wpsi = w(2);
ws = w(3:4);
wkappa = w(5);
ey = -sin(wpsi) * (s(1) - ws(1)) + cos(wpsi) * (s(2) - ws(2));
epsi = mod(psi - wpsi + pi, 2*pi) - pi;
end

== matlab function s06_sig_template/Maneuver1/Create Maneuver ==
  data: type input; vmax input; xref input; P_track parameter; P_cpseq parameter; maneuver output Bus: DRIVEMANEUVER size=1
function maneuver = create_maneuver(type, vmax, xref, P_track, P_cpseq)
%#codegen

track = P_track.center;

maneuver = struct( ...
    'vmax', vmax, ... 
    'type', type, ...
    'xref', xref, ...
    'lapCount', uint32(0), ...
    'disableLaneMonitor', false, ...
    'isnew', true, ...
    'breakslen', track.breakslen, ...
    'points', track.points, ...
    'coefs', track.coefs, ...
    'segments', zeros(1, length(track.points), 'uint32'), ...
    'periodic', true, ...
    'cpseq', P_cpseq);
end

== matlab function s06_sig_template/Localization/Locate/ObsSpline/wx derivative ==
  data: wx input; wxm1 input; xe input; wxd output; P_dt parameter
function wxd  = wx2wv(wx, wxm1, xe, P_dt)
wxd = single(0);
if wxm1 > -1
    wxd = (mod(wx - wxm1 + 0.5 * xe, xe) - 0.5 * xe) / P_dt;
end
end

== matlab function s06_sig_template/Maneuver0/Create Maneuver ==
  data: type input; vmax input; xref input; P_track parameter; P_cpseq parameter; maneuver output Bus: DRIVEMANEUVER size=1
function maneuver = create_maneuver(type, vmax, xref, P_track, P_cpseq)
%#codegen

track = P_track.center;

maneuver = struct( ...
    'vmax', vmax, ... 
    'type', type, ...
    'xref', xref, ...
    'lapCount', uint32(0), ...
    'disableLaneMonitor', false, ...
    'isnew', true, ...
    'breakslen', track.breakslen, ...
    'points', track.points, ...
    'coefs', track.coefs, ...
    'segments', zeros(1, length(track.points), 'uint32'), ...
    'periodic', true, ...
    'cpseq', P_cpseq);
end

== matlab function s06_sig_template/Localization/Locate/ObsSpline/Reference and Deviations1 ==
  data: wxe output; s input; psi input; widxkm1 input int32; spline input; P_c_spline_range parameter; w output; widx output; ey output; epsi output
function [ wxe, w, widx, ey, epsi ] = fcn(s, psi, widxkm1, spline, P_c_spline_range)
%#codegen
wxe = spline.points(1, spline.breakslen);
if widxkm1 < int32(1)
    % first call
    irangemin = int32(1);
    irangemax = int32(spline.breakslen);
else
    irangemin = widxkm1 - P_c_spline_range;
    irangemax = widxkm1 + P_c_spline_range;
end
[ w , widx ] = mbc_spline_get_reference(s, spline.breakslen, spline.points, spline.coefs, spline.periodic, 0, 0, irangemin, irangemax);
wpsi = w(2);
ws = w(3:4);
ey = -sin(wpsi) * (s(1) - ws(1)) + cos(wpsi) * (s(2) - ws(2));
epsi = mod(psi - wpsi + pi, 2*pi) - pi;
end

== matlab function s06_sig_template/Localization/Locate/ObsSpline/Reference and Deviations2 ==
  data: wxe output; s input; psi input; widxkm1 input int32; spline input; P_c_spline_range parameter; w output; widx output; ey output; epsi output
function [ wxe, w, widx, ey, epsi ] = fcn(s, psi, widxkm1, spline, P_c_spline_range)
%#codegen
wxe = spline.points(1, spline.breakslen);
if widxkm1 < int32(1)
    % first call
    irangemin = int32(1);
    irangemax = int32(spline.breakslen);
else
    irangemin = widxkm1 - P_c_spline_range;
    irangemax = widxkm1 + P_c_spline_range;
end
[ w , widx ] = mbc_spline_get_reference(s, spline.breakslen, spline.points, spline.coefs, spline.periodic, 0, 0, irangemin, irangemax);
wpsi = w(2);
ws = w(3:4);
ey = -sin(wpsi) * (s(1) - ws(1)) + cos(wpsi) * (s(2) - ws(2));
epsi = mod(psi - wpsi + pi, 2*pi) - pi;
end
